simulink model "PMSM_HF_4_2019b"  (R2019b)
settings: Solver=VariableStepAuto  StartTime=0.0  StopTime=10.0  RelTol=1e-3
libraries: powerlib x5, simulink x1, dsparch4 x1
settings Model: Creator=Administrator  LastModifiedBy=Administrator

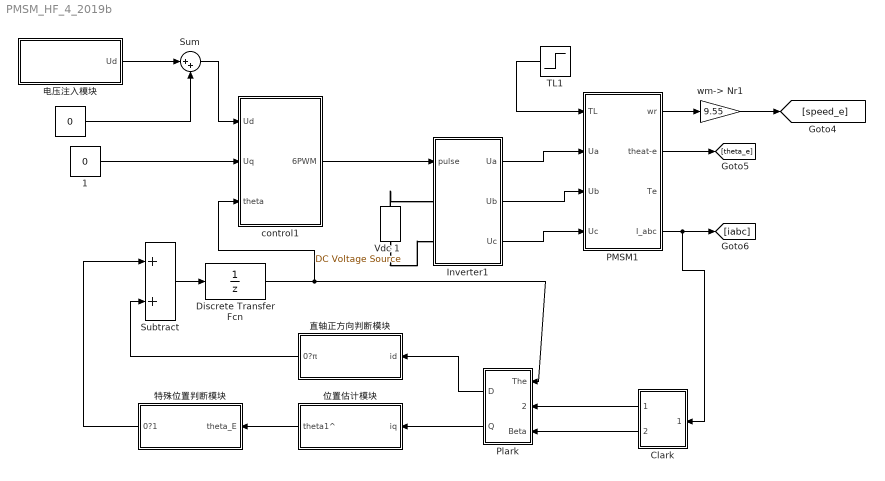
== system PMSM_HF_4_2019b ==
  "   " : Constant  Value=0
  "   1" : Constant  Value=0
  Clark : Subsystem
  Discrete Transfer Fcn : DiscreteTransferFcn  Denominator=[1 0]
  Inverter1 : Subsystem
  PMSM1 : Subsystem  mask{Ld=0.0052, R=0.33, Lq=0.0174, kf=0.646, p=2, F=0, J=0.008}
  Plark : Subsystem
  Subtract : Sum
  Sum : Sum  Inputs=|++
  TL1 : Step  Time=0.05  After=0  SampleTime=0
  Vdc 1 : powerlib/Electrical Sources/DC Voltage Source  Amplitude=311  Measurements=None
      settings: SourceProductName=Simscape Electrical
  control1 : Subsystem
  wm-> Nr1 : Gain  Gain=9.55
  位置估计模块 : Subsystem
  特殊位置判断模块 : Subsystem
  电压注入模块 : Subsystem
  直轴正方向判断模块 : Subsystem
  wires:
  位置估计模块/1(theta1^) -> 特殊位置判断模块/1(theta_E)
  Clark/2(Beta) -> Plark/3(Beta)
  Plark/2(Q) -> 位置估计模块/1(iq)
  "   "/1 -> Sum/2
  特殊位置判断模块/1(0?1) -> Subtract/1
  Plark/1(D) -> 直轴正方向判断模块/1(id)
  PMSM1/1(wr) -> wm-> Nr1/1
  PMSM1/4(I_abc) -> Clark/1(ABC), [iabc]
  Inverter1/1(Ua) -> PMSM1/2(Ua)
  PMSM1/2(theat-e) -> [theta_e]
  Inverter1/3(Uc) -> PMSM1/4(Uc)
  Subtract/1 -> Discrete Transfer Fcn/1
  Clark/1(Alpha) -> Plark/2(Alpha)
  Sum/1 -> control1/1(Ud)
  Discrete Transfer Fcn/1 -> control1/3(theta), Plark/1(The)
  wm-> Nr1/1 -> [speed_e]
  TL1/1 -> PMSM1/1(TL)
  电压注入模块/1(Ud) -> Sum/1
  "   1"/1 -> control1/2(Uq)
  Inverter1/2(Ub) -> PMSM1/3(Ub)
  control1/1(6PWM) -> Inverter1/1(pulse)
  直轴正方向判断模块/1(0?π) -> Subtract/2
  connections:
  Vdc 1/LConn1 -- Inverter1/LConn2
  Vdc 1/RConn1 -- Inverter1/LConn1

== system PMSM_HF_4_2019b/Clark ==
  ABC : Inport
  alpha : Fcn  Expr=(u(1)-0.5*(u(2)+u(3)))*2/3
  beta : Fcn  Expr=sqrt(3)/2*(u(2)-u(3))*2/3
  Alpha : Outport
  Beta : Outport  Port=2
  wires:
  alpha/1 -> Alpha/1
  ABC/1 -> beta/1, alpha/1
  beta/1 -> Beta/1

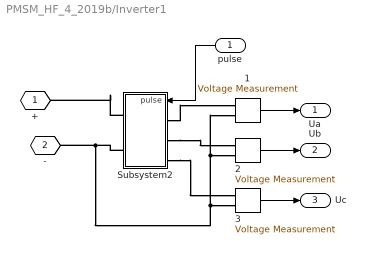
== system PMSM_HF_4_2019b/Inverter1 ==
  pulse : Inport
  1 : powerlib/Measurements/Voltage Measurement  PhasorSimulation=off  OutputType=Complex  PSBequivalent=0
      settings: SourceProductName=Simscape Electrical
  2 : powerlib/Measurements/Voltage Measurement  PhasorSimulation=off  OutputType=Complex  PSBequivalent=0
      settings: SourceProductName=Simscape Electrical
  3 : powerlib/Measurements/Voltage Measurement  PhasorSimulation=off  OutputType=Complex  PSBequivalent=0
      settings: SourceProductName=Simscape Electrical
  Subsystem2 : Subsystem
  + : PMIOPort  Tag=PMCPort  Side=Left
  - : PMIOPort  Tag=PMCPort  Port=2  Side=Left
  Ua : Outport
  Ub : Outport  Port=2
  Uc : Outport  Port=3
  wires:
  3/1 -> Uc/1
  2/1 -> Ub/1
  1/1 -> Ua/1
  pulse/1 -> Subsystem2/1(pulse)
  connections:
  Subsystem2/LConn1 -- 1/LConn1
  -/RConn1 -- Subsystem2/RConn2 -- 3/LConn2 -- 2/LConn2 -- 1/LConn2
  Subsystem2/LConn2 -- 2/LConn1
  Subsystem2/LConn3 -- 3/LConn1
  Subsystem2/RConn1 -- +/RConn1

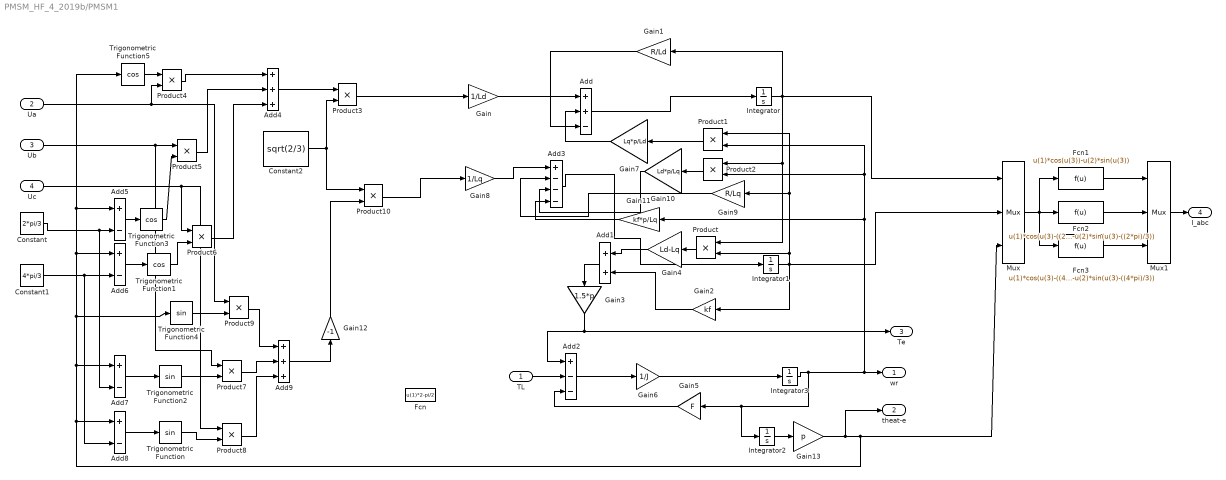
== system PMSM_HF_4_2019b/PMSM1 ==
  TL : Inport
  Ua : Inport  Port=2
  Ub : Inport  Port=3
  Uc : Inport  Port=4
  Add : Sum  Inputs=++-
  Add1 : Sum
  Add2 : Sum  Inputs=+--
  Add3 : Sum  Inputs=+---
  Add4 : Sum  Inputs=+++
  Add{5..8} (4 alike) : Sum  Inputs=+-
  Add9 : Sum  Inputs=+++
  Constant : Constant  Value=2*pi/3
  Constant1 : Constant  Value=4*pi/3
  Constant2 : Constant  Value=sqrt(2/3)
  Fcn : Fcn  Expr=u(1)*2-pi/2
  Fcn1 : Fcn  Expr=u(1)*cos(u(3))-u(2)*sin(u(3))
  Fcn2 : Fcn  Expr=u(1)*cos(u(3)-((2*pi)/3))-u(2)*sin(u(3)-((2*pi)/3))
  Fcn3 : Fcn  Expr=u(1)*cos(u(3)-((4*pi)/3))-u(2)*sin(u(3)-((4*pi)/3))
  Gain : Gain  Gain=1/Ld
  Gain1 : Gain  Gain=R/Ld
  Gain10 : Gain  Gain=Ld*p/Lq
  Gain11 : Gain  Gain=kf*p/Lq
  Gain12 : Gain  Gain=-1
  Gain13 : Gain  Gain=p
  Gain2 : Gain  Gain=kf
  Gain3 : Gain  Gain=1.5*p
  Gain4 : Gain  Gain=Ld-Lq
  Gain5 : Gain  Gain=F
  Gain6 : Gain  Gain=1/J
  Gain7 : Gain  Gain=Lq*p/Ld
  Gain8 : Gain  Gain=1/Lq
  Gain9 : Gain  Gain=R/Lq
  Integrator{,1..3} (4 alike) : Integrator
  Mux : Mux  Inputs=3
  Mux1 : Mux  Inputs=3
  Product{,1..10} (11 alike) : Product  RndMeth=Zero
  Trigonometric Function : Trigonometry
  Trigonometric Function1 : Trigonometry  Operator=cos
  Trigonometric Function2 : Trigonometry
  Trigonometric Function3 : Trigonometry  Operator=cos
  Trigonometric Function4 : Trigonometry
  Trigonometric Function5 : Trigonometry  Operator=cos
  wr : Outport
  theat-e : Outport  Port=2
  Te : Outport  Port=3
  I_abc : Outport  Port=4
  wires:
  Add3/1 -> Integrator1/1
  Gain11/1 -> Add3/4
  Gain10/1 -> Add3/3
  Product2/1 -> Gain10/1
  Gain9/1 -> Add3/2
  Gain8/1 -> Add3/1
  Add/1 -> Integrator/1
  Gain7/1 -> Add/2
  Product1/1 -> Gain7/1
  Gain6/1 -> Integrator3/1
  Add2/1 -> Gain6/1
  Gain5/1 -> Add2/3
  TL/1 -> Add2/2
  Integrator3/1 -> wr/1, Product1/2, Product2/2, Gain11/1, Gain5/1, Integrator2/1
  Gain3/1 -> Add2/1, Te/1
  Add1/1 -> Gain3/1
  Gain2/1 -> Add1/2
  Gain4/1 -> Add1/1
  Product/1 -> Gain4/1
  Gain1/1 -> Add/3
  Integrator1/1 -> Product/2, Product1/1, Gain9/1, Gain2/1, Mux/2
  Integrator/1 -> Gain1/1, Product/1, Product2/1, Mux/1
  Gain/1 -> Add/1
  Constant2/1 -> Product3/2, Product10/1
  Add4/1 -> Product3/1
  Product3/1 -> Gain/1
  Constant/1 -> Add5/2, Add7/2
  Add5/1 -> Trigonometric Function3/1
  Constant1/1 -> Add6/2, Add8/2
  Add6/1 -> Trigonometric Function1/1
  Trigonometric Function5/1 -> Product4/1
  Ua/1 -> Product4/2, Product9/1
  Product4/1 -> Add4/1
  Ub/1 -> Product5/1, Product7/1
  Trigonometric Function3/1 -> Product5/2
  Product5/1 -> Add4/2
  Uc/1 -> Product6/1, Product8/1
  Trigonometric Function1/1 -> Product6/2
  Product6/1 -> Add4/3
  Add7/1 -> Trigonometric Function2/1
  Add8/1 -> Trigonometric Function/1
  Trigonometric Function2/1 -> Product7/2
  Trigonometric Function/1 -> Product8/2
  Trigonometric Function4/1 -> Product9/2
  Product9/1 -> Add9/1
  Product7/1 -> Add9/2
  Product8/1 -> Add9/3
  Add9/1 -> Gain12/1
  Gain12/1 -> Product10/2
  Product10/1 -> Gain8/1
  Gain13/1 -> Add8/1, Add7/1, Trigonometric Function5/1, Add5/1, Add6/1, Trigonometric Function4/1, Mux/3, theat-e/1
  Fcn3/1 -> Mux1/3
  Fcn2/1 -> Mux1/2
  Fcn1/1 -> Mux1/1
  Mux/1 -> Fcn2/1, Fcn1/1, Fcn3/1
  Mux1/1 -> I_abc/1
  Integrator2/1 -> Gain13/1

== system PMSM_HF_4_2019b/Plark ==
  The : Inport
  Alpha : Inport  Port=2
  Beta : Inport  Port=3
  Mux : Mux  Inputs=3
  d : Fcn  Expr=u(1)*cos(u(3))+u(2)*sin(u(3))
  q : Fcn  Expr=-u(1)*sin(u(3))+u(2)*cos(u(3))
  D : Outport
  Q : Outport  Port=2
  wires:
  d/1 -> D/1
  Beta/1 -> Mux/2
  The/1 -> Mux/3
  Alpha/1 -> Mux/1
  Mux/1 -> q/1, d/1
  q/1 -> Q/1

== system PMSM_HF_4_2019b/control1 ==
  Ud : Inport
  Uq : Inport  Port=2
  theta : Inport  Port=3
  Anti_Plark : Subsystem
  SVPWM : Subsystem
  6PWM : Outport
  wires:
  SVPWM/1(pulse) -> 6PWM/1
  Ud/1 -> Anti_Plark/1(D)
  Anti_Plark/1(Alpha) -> SVPWM/1(Ualfa)
  Anti_Plark/2(Beta) -> SVPWM/2(Ubeta)
  Uq/1 -> Anti_Plark/2(Q)
  theta/1 -> Anti_Plark/3(The)

== system PMSM_HF_4_2019b/位置估计模块 ==
  iq : Inport
  0-100ms : Step  Time=0.1  Before=1  After=0  SampleTime=0
  1/J : Gain  Gain=1/0.008
  Analog Filter Design : dsparch4/Analog Filter Design  method=Butterworth  filttype=Lowpass  N=1  Wlo=942  Whi=80  Rp=2  Rs=40
  Integrator2 : Integrator
  Sine Wave1 : Sin  Frequency=6280  SampleTime=0
  正向电压脉冲1 : Product  Inputs=3
  theta1^ : Outport
  wires:
  Sine Wave1/1 -> 正向电压脉冲1/2
  iq/1 -> 正向电压脉冲1/1
  0-100ms/1 -> 正向电压脉冲1/3
  正向电压脉冲1/1 -> Analog Filter Design/1
  1/J/1 -> Integrator2/1
  Analog Filter Design/1 -> 1/J/1
  Integrator2/1 -> theta1^/1

== system PMSM_HF_4_2019b/特殊位置判断模块 ==
  theta_E : Inport
  25ms时 : Step  Time=0.025  SampleTime=0
  Abs : Abs
  Relational Operator : RelationalOperator  Operator=<=  OutDataTypeStr=boolean  RndMeth=Simplest
  Triggered Subsystem : Subsystem  TreatAsAtomicUnit=on
  估计位置初始值 : Constant
  正向电压脉冲1 : Product  Inputs=3
  误差值 : Constant  Value=0.05
  0?1 : Outport
  wires:
  theta_E/1 -> Triggered Subsystem/1(In1)
  Triggered Subsystem/1(Out1) -> Abs/1
  Abs/1 -> Relational Operator/1
  误差值/1 -> Relational Operator/2
  Relational Operator/1 -> 正向电压脉冲1/2
  正向电压脉冲1/1 -> 0?1/1
  25ms时/1 -> Triggered Subsystem/Trigger, 正向电压脉冲1/1
  估计位置初始值/1 -> 正向电压脉冲1/3

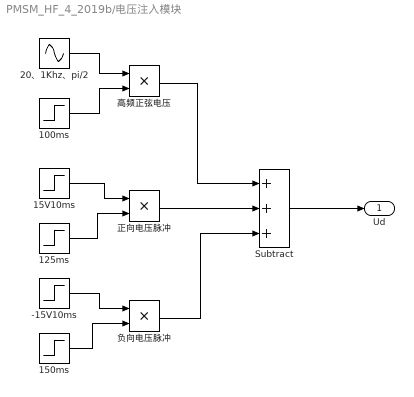
== system PMSM_HF_4_2019b/电压注入模块 ==
  -15V10ms : Step  Time=0.16  Before=-15  After=0  SampleTime=0
  100ms : Step  Time=0.1  Before=1  After=0  SampleTime=0
  125ms : Step  Time=0.125  SampleTime=0
  150ms : Step  Time=0.15  SampleTime=0
  15V10ms : Step  Time=0.135  Before=15  After=0  SampleTime=0
  20、1Khz、pi/2 : Sin  Amplitude=20  Frequency=6280  Phase=pi/2  SampleTime=0
  Subtract : Sum  Inputs=+++
  正向电压脉冲 : Product
  负向电压脉冲 : Product
  高频正弦电压 : Product
  Ud : Outport
  wires:
  20、1Khz、pi/2/1 -> 高频正弦电压/1
  100ms/1 -> 高频正弦电压/2
  高频正弦电压/1 -> Subtract/1
  15V10ms/1 -> 正向电压脉冲/1
  125ms/1 -> 正向电压脉冲/2
  -15V10ms/1 -> 负向电压脉冲/1
  150ms/1 -> 负向电压脉冲/2
  正向电压脉冲/1 -> Subtract/2
  负向电压脉冲/1 -> Subtract/3
  Subtract/1 -> Ud/1

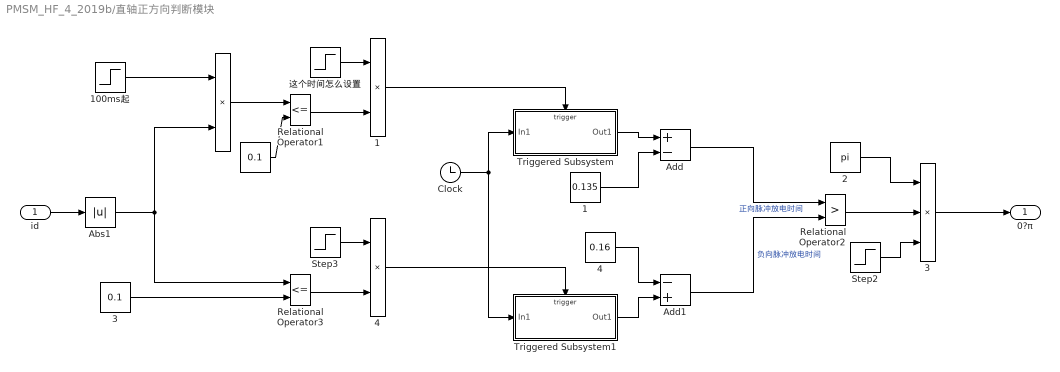
== system PMSM_HF_4_2019b/直轴正方向判断模块 ==
  id : Inport
  " " : Constant  Value=0.1
  "  " : Product
  "  1" : Product
  "  3" : Product  Inputs=3
  "  4" : Product
  " 1" : Constant  Value=0.135
  " 2" : Constant  Value=pi
  " 3" : Constant  Value=0.1
  " 4" : Constant  Value=0.16
  100ms起 : Step  Time=0.1  SampleTime=0
  Abs1 : Abs
  Add : Sum  Inputs=+-
  Add1 : Sum  Inputs=-+
  Clock : Clock
  Relational Operator1 : RelationalOperator  Operator=<=  OutDataTypeStr=boolean  RndMeth=Simplest
  Relational Operator2 : RelationalOperator  Operator=>  OutDataTypeStr=boolean  RndMeth=Simplest
  Relational Operator3 : RelationalOperator  Operator=<=  OutDataTypeStr=boolean  RndMeth=Simplest
  Step2 : Step  Time=0.175  SampleTime=0
  Step3 : Step  SampleTime=0
  Triggered Subsystem : Subsystem  TreatAsAtomicUnit=on
  Triggered Subsystem1 : Subsystem  TreatAsAtomicUnit=on
  这个时间怎么设置 : Step  Time=0.135  SampleTime=0
  0?π : Outport
  wires:
  id/1 -> Abs1/1
  100ms起/1 -> "  "/1
  "  "/1 -> Relational Operator1/1
  " "/1 -> Relational Operator1/2
  这个时间怎么设置/1 -> "  1"/1
  "  1"/1 -> Triggered Subsystem/Trigger
  Relational Operator1/1 -> "  1"/2
  " 1"/1 -> Add/2
  " 2"/1 -> "  3"/1
  Relational Operator2/1 -> "  3"/2
  Step2/1 -> "  3"/3
  "  3"/1 -> 0?π/1
  Relational Operator3/1 -> "  4"/2
  Step3/1 -> "  4"/1
  " 3"/1 -> Relational Operator3/2
  Abs1/1 -> Relational Operator3/1, "  "/2
  "  4"/1 -> Triggered Subsystem1/Trigger
  Triggered Subsystem/1(Out1) -> Add/1
  Add/1 -> Relational Operator2/1  "正向脉冲放电时间"
  " 4"/1 -> Add1/1
  Triggered Subsystem1/1(Out1) -> Add1/2
  Add1/1 -> Relational Operator2/2  "负向脉冲放电时间"
  Clock/1 -> Triggered Subsystem1/1(In1), Triggered Subsystem/1(In1)

== system PMSM_HF_4_2019b/Inverter1/Subsystem2 ==
  pulse : Inport
  Universal Bridge : powerlib/Power Electronics/Universal Bridge  Arms=3  SnubberResistance=1e5  SnubberCapacitance=inf  Device=IGBT / Diodes  Ron=1e-3  Lon=0  ForwardVoltages="[  0  0  ]"  ForwardVoltage=0  GTOparameters=[ 10e-6 , 20e-6 ]  IGBTparameters=[ 1e-6 , 2e-6 ]  Measurements=None  Measurements_2=None  converterType=Rectifier
      settings: SourceProductName=Simscape Electrical
  Ua : PMIOPort  Tag=PMCPort  Side=Left
  Ub : PMIOPort  Tag=PMCPort  Port=2  Side=Left
  Uc : PMIOPort  Tag=PMCPort  Port=3  Side=Left
  + : PMIOPort  Tag=PMCPort  Port=4  Side=Right
  - : PMIOPort  Tag=PMCPort  Port=5  Side=Right
  wires:
  pulse/1 -> Universal Bridge/1
  connections:
  Universal Bridge/LConn1 -- Ua/RConn1
  Universal Bridge/LConn2 -- Ub/RConn1
  Universal Bridge/LConn3 -- Uc/RConn1
  +/RConn1 -- Universal Bridge/RConn1
  -/RConn1 -- Universal Bridge/RConn2

== system PMSM_HF_4_2019b/control1/Anti_Plark ==
  D : Inport
  Q : Inport  Port=2
  The : Inport  Port=3
  Mux : Mux  Inputs=3
  alpha : Fcn  Expr=u(1)*cos(u(3))-u(2)*sin(u(3))
  beta : Fcn  Expr=u(1)*sin(u(3))+u(2)*cos(u(3))
  Alpha : Outport
  Beta : Outport  Port=2
  wires:
  beta/1 -> Beta/1
  Mux/1 -> alpha/1, beta/1
  D/1 -> Mux/1
  The/1 -> Mux/3
  Q/1 -> Mux/2
  alpha/1 -> Alpha/1

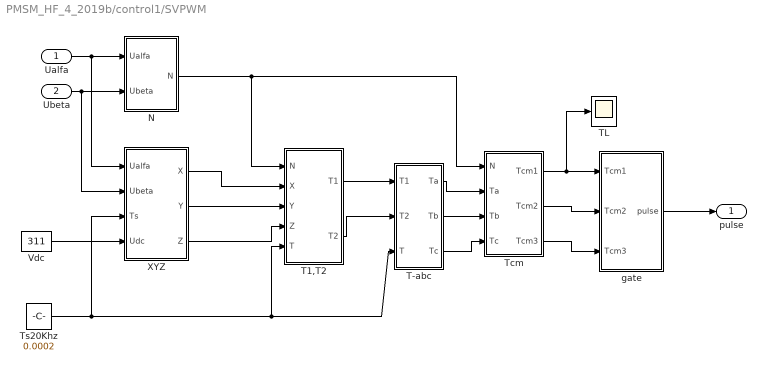
== system PMSM_HF_4_2019b/control1/SVPWM ==
  Ualfa : Inport
  Ubeta : Inport  Port=2
  N : Subsystem
  T-abc : Subsystem
  T1,T2 : Subsystem
  TL : Scope
  Tcm : Subsystem
  Ts20Khz : Constant  Value=0.0002  SampleTime=-1
  Vdc : Constant  Value=311
  XYZ : Subsystem
  gate : Subsystem
  pulse : Outport
  wires:
  Tcm/3(Tcm3) -> gate/3(Tcm3)
  Tcm/2(Tcm2) -> gate/2(Tcm2)
  Vdc/1 -> XYZ/4(Udc)
  Ubeta/1 -> XYZ/2(Ubeta), N/2(Ubeta)
  Ualfa/1 -> XYZ/1(Ualfa), N/1(Ualfa)
  gate/1(pulse) -> pulse/1
  Ts20Khz/1 -> XYZ/3(Ts), T-abc/3(T), T1,T2/5(T)
  N/1(N) -> Tcm/1(N), T1,T2/1(N)
  XYZ/3(Z) -> T1,T2/4(Z)
  XYZ/1(X) -> T1,T2/2(X)
  XYZ/2(Y) -> T1,T2/3(Y)
  T1,T2/2(T2) -> T-abc/2(T2)
  T1,T2/1(T1) -> T-abc/1(T1)
  T-abc/3(Tc) -> Tcm/4(Tc)
  T-abc/1(Ta) -> Tcm/2(Ta)
  T-abc/2(Tb) -> Tcm/3(Tb)
  Tcm/1(Tcm1) -> TL/1, gate/1(Tcm1)

== system PMSM_HF_4_2019b/特殊位置判断模块/Triggered Subsystem ==
  In1 : Inport
  Trigger : TriggerPort  VariantControl=Variant
  Out1 : Outport
  wires:
  In1/1 -> Out1/1

== system PMSM_HF_4_2019b/直轴正方向判断模块/Triggered Subsystem ==
  In1 : Inport
  Trigger : TriggerPort  VariantControl=Variant
  Out1 : Outport
  wires:
  In1/1 -> Out1/1

== system PMSM_HF_4_2019b/直轴正方向判断模块/Triggered Subsystem1 ==
  In1 : Inport
  Trigger : TriggerPort  VariantControl=Variant
  Out1 : Outport
  wires:
  In1/1 -> Out1/1

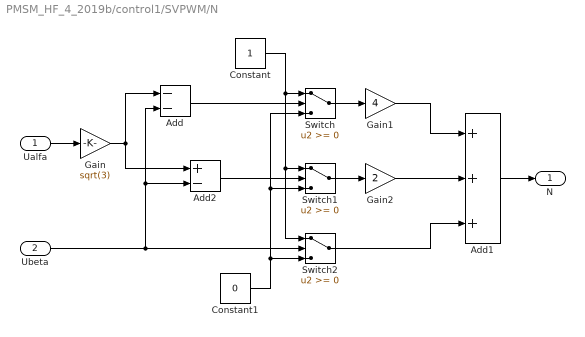
== system PMSM_HF_4_2019b/control1/SVPWM/N ==
  Ualfa : Inport
  Ubeta : Inport  Port=2
  Add : Sum  Inputs=--
  Add1 : Sum  Inputs=+++
  Add2 : Sum  Inputs=+-
  Constant : Constant
  Constant1 : Constant  Value=0
  Gain : Gain  Gain=sqrt(3)
  Gain1 : Gain  Gain=4
  Gain2 : Gain  Gain=2
  Switch : Switch
  Switch1 : Switch
  Switch2 : Switch
  N : Outport
  wires:
  Constant1/1 -> Switch2/3, Switch1/3, Switch/3
  Constant/1 -> Switch/1, Switch1/1, Switch2/1
  Gain2/1 -> Add1/2
  Switch1/1 -> Gain2/1
  Add2/1 -> Switch1/2
  Switch2/1 -> Add1/3
  Gain1/1 -> Add1/1
  Ubeta/1 -> Add2/2, Add/2, Switch2/2
  Gain/1 -> Add2/1, Add/1
  Add/1 -> Switch/2
  Switch/1 -> Gain1/1
  Add1/1 -> N/1
  Ualfa/1 -> Gain/1

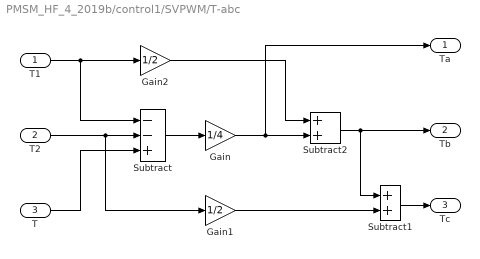
== system PMSM_HF_4_2019b/control1/SVPWM/T-abc ==
  T1 : Inport
  T2 : Inport  Port=2
  T : Inport  Port=3
  Gain : Gain  Gain=1/4
  Gain1 : Gain  Gain=1/2
  Gain2 : Gain  Gain=1/2
  Subtract : Sum  Inputs=--+
  Subtract1 : Sum
  Subtract2 : Sum
  Ta : Outport
  Tb : Outport  Port=2
  Tc : Outport  Port=3
  wires:
  Gain1/1 -> Subtract1/2
  Subtract1/1 -> Tc/1
  Subtract2/1 -> Subtract1/1, Tb/1
  Gain2/1 -> Subtract2/1
  Gain/1 -> Subtract2/2, Ta/1
  Subtract/1 -> Gain/1
  T/1 -> Subtract/3
  T1/1 -> Gain2/1, Subtract/1
  T2/1 -> Gain1/1, Subtract/2

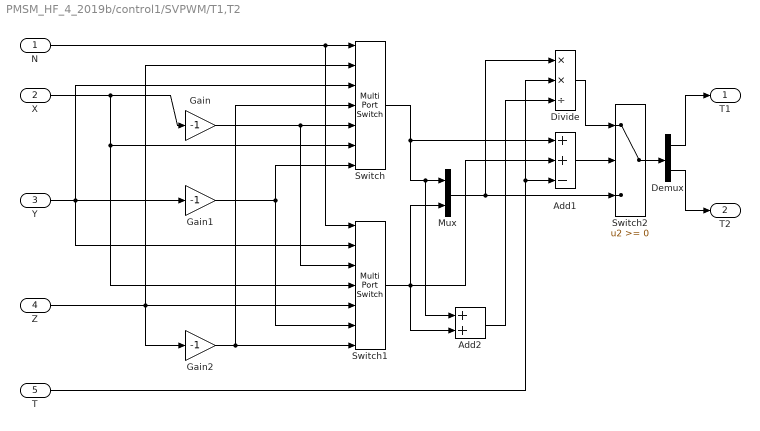
== system PMSM_HF_4_2019b/control1/SVPWM/T1,T2 ==
  N : Inport
  X : Inport  Port=2
  Y : Inport  Port=3
  Z : Inport  Port=4
  T : Inport  Port=5
  Add1 : Sum  Inputs=++-
  Add2 : Sum
  Demux : Demux  Outputs=2
  Divide : Product  Inputs=**/
  Gain : Gain  Gain=-1
  Gain1 : Gain  Gain=-1
  Gain2 : Gain  Gain=-1
  Mux : Mux  Inputs=2
  Switch : MultiPortSwitch  Inputs=6
  Switch1 : MultiPortSwitch  Inputs=6
  Switch2 : Switch
  T1 : Outport
  T2 : Outport  Port=2
  wires:
  N/1 -> Switch1/1, Switch/1
  Add2/1 -> Divide/3
  Divide/1 -> Switch2/1
  T/1 -> Divide/2, Add1/3
  Add1/1 -> Switch2/2
  Demux/2 -> T2/1
  Demux/1 -> T1/1
  Switch2/1 -> Demux/1
  Mux/1 -> Switch2/3, Divide/1
  Switch1/1 -> Add2/2, Add1/2, Mux/2
  Switch/1 -> Add2/1, Mux/1, Add1/1
  Gain1/1 -> Switch/7, Switch1/6
  Gain2/1 -> Switch1/7, Switch/4
  Gain/1 -> Switch1/3, Switch/5
  X/1 -> Switch/6, Switch1/4, Gain/1
  Z/1 -> Gain2/1, Switch1/5, Switch/2
  Y/1 -> Switch1/2, Gain1/1, Switch/3

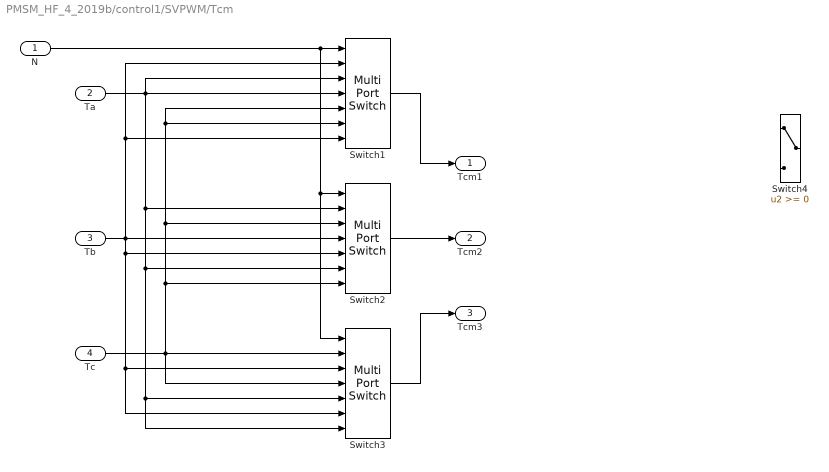
== system PMSM_HF_4_2019b/control1/SVPWM/Tcm ==
  N : Inport
  Ta : Inport  Port=2
  Tb : Inport  Port=3
  Tc : Inport  Port=4
  Switch1 : MultiPortSwitch  Inputs=6
  Switch2 : MultiPortSwitch  Inputs=6
  Switch3 : MultiPortSwitch  Inputs=6
  Switch4 : Switch
  Tcm1 : Outport
  Tcm2 : Outport  Port=2
  Tcm3 : Outport  Port=3
  wires:
  N/1 -> Switch3/1, Switch2/1, Switch1/1
  Ta/1 -> Switch3/7, Switch3/5, Switch2/6, Switch2/2, Switch1/3, Switch1/4
  Tc/1 -> Switch2/7, Switch1/6, Switch1/5, Switch2/3, Switch3/4, Switch3/2
  Tb/1 -> Switch1/7, Switch1/2, Switch3/6, Switch3/3, Switch2/5, Switch2/4
  Switch1/1 -> Tcm1/1
  Switch3/1 -> Tcm3/1
  Switch2/1 -> Tcm2/1

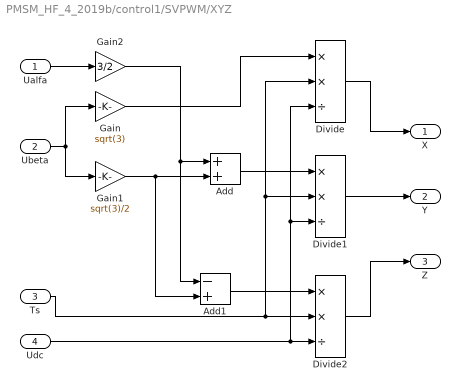
== system PMSM_HF_4_2019b/control1/SVPWM/XYZ ==
  Ualfa : Inport
  Ubeta : Inport  Port=2
  Ts : Inport  Port=3
  Udc : Inport  Port=4
  Add : Sum
  Add1 : Sum  Inputs=-+
  Divide : Product  Inputs=**/
  Divide1 : Product  Inputs=**/
  Divide2 : Product  Inputs=**/
  Gain : Gain  Gain=sqrt(3)
  Gain1 : Gain  Gain=sqrt(3)/2
  Gain2 : Gain  Gain=3/2
  X : Outport
  Y : Outport  Port=2
  Z : Outport  Port=3
  wires:
  Add1/1 -> Divide2/1
  Gain2/1 -> Add/1, Add1/1
  Gain1/1 -> Add1/2, Add/2
  Add/1 -> Divide1/1
  Gain/1 -> Divide/1
  Ualfa/1 -> Gain2/1
  Ubeta/1 -> Gain1/1, Gain/1
  Udc/1 -> Divide/3, Divide1/3, Divide2/3
  Ts/1 -> Divide/2, Divide1/2, Divide2/2
  Divide2/1 -> Z/1
  Divide/1 -> X/1
  Divide1/1 -> Y/1

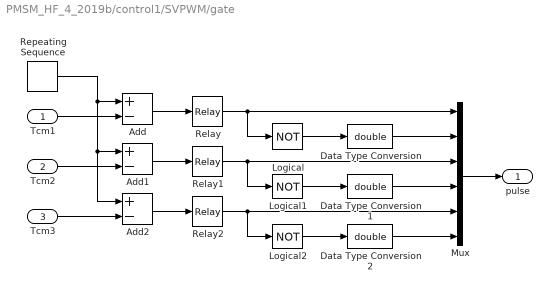
== system PMSM_HF_4_2019b/control1/SVPWM/gate ==
  Tcm1 : Inport
  Tcm2 : Inport  Port=2
  Tcm3 : Inport  Port=3
  Add : Sum  Inputs=+-
  Add1 : Sum  Inputs=+-
  Add2 : Sum  Inputs=+-
  Data Type Conversion : DataTypeConversion  OutDataTypeStr=double
  Data Type Conversion1 : DataTypeConversion  OutDataTypeStr=double
  Data Type Conversion2 : DataTypeConversion  OutDataTypeStr=double
  Logical : Logic  Operator=NOT  AllPortsSameDT=off  OutDataTypeStr=boolean
  Logical1 : Logic  Operator=NOT  AllPortsSameDT=off  OutDataTypeStr=boolean
  Logical2 : Logic  Operator=NOT  AllPortsSameDT=off  OutDataTypeStr=boolean
  Mux : Mux  Inputs=6
  Relay : Relay
  Relay1 : Relay
  Relay2 : Relay
  Repeating Sequence : simulink/Sources/Repeating Sequence  rep_seq_t=[0 0.00005 0.0001]  rep_seq_y=[0 0.0001 0]
  pulse : Outport
  wires:
  Mux/1 -> pulse/1
  Logical2/1 -> Data Type Conversion2/1
  Data Type Conversion2/1 -> Mux/6
  Logical1/1 -> Data Type Conversion1/1
  Data Type Conversion1/1 -> Mux/4
  Logical/1 -> Data Type Conversion/1
  Data Type Conversion/1 -> Mux/2
  Relay2/1 -> Logical2/1, Mux/5
  Relay1/1 -> Logical1/1, Mux/3
  Relay/1 -> Logical/1, Mux/1
  Add/1 -> Relay/1
  Add1/1 -> Relay1/1
  Add2/1 -> Relay2/1
  Repeating Sequence/1 -> Add/1, Add1/1, Add2/1
  Tcm3/1 -> Add2/2
  Tcm2/1 -> Add1/2
  Tcm1/1 -> Add/2
